simulink model "trabajo"  (R2021b)
settings: Solver=VariableStepAuto  StartTime=0.0  StopTime=1000  RelTol=1e-3
settings Model: Creator=david  LastModifiedBy=david

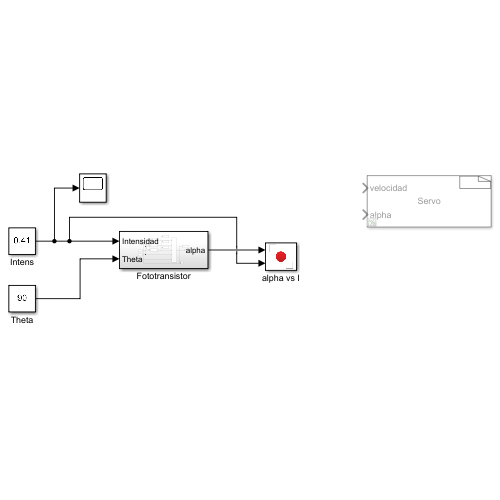
[thumbnail: Simulink's stored preview of the top-level diagram]
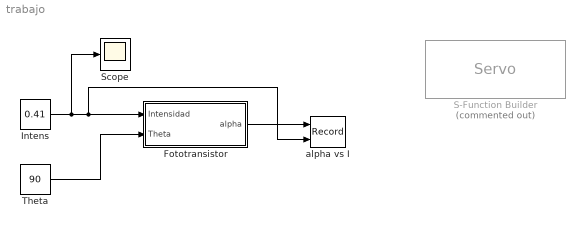
== system trabajo ==
  Fototransistor : Subsystem
  Intens : Constant  Value=0.41
  S-Function Builder : S-Function  Commented=on  FunctionName=Servo  SFunctionDeploymentMode=off  EnableBusSupport=off  mask(S-Function Builder){}
      mask help: Simulink:masks:SFunctionBuilder_MD
      mask init:
      | val = [[.9  0.75 0.75 1 1 .9 .9 1]',[1 1 0.75 0.75 .9 .9 1 .9]'];try , sys = get_param(gcb,'SfunBuilderFcnName');if isempty(sys), sys = get_param(gcb,'FunctionName'); end,catch, sys = get_param(gcb,'FunctionName'); end
      settings: CopyFcn=set_param(gcbh,'LinkStatus','none')  OpenFcn=sfunctionwizard(gcbh)
      mask Display: plot(val(:,1),val(:,2)),disp(sys),port_label('input',1,'velocidad'),port_label('input',2,'alpha')
  Scope : Scope
  Theta : Constant  Value=90
  alpha vs I : Record  FileSettingsInternal="{\"entries\":[{\"content\":{\"excelSettings\":{\"content\":{},\"type\":\"Streamout.ExcelSettings\"}},\"type\":\"Streamout.FileSettingStorage\",\"uuid\":\"fbcb0ebc-f8fb-453b-844a-01a15ffa13b0\"}],\"packageUris\":[\"http://schema.mathworks.com/mf0/streamout_blocks/R2020a\"],\"version\":\"1.0\"}"  Layout=[1 1]  SignalsInternal="{\"entries\":[{\"content\":{\"signals\":[{\"content\":{\"blockPath\":[\"trabajo/alpha vs I\"],\"channel\":[],\"dimensions\":[1],\"domain\":\"trabajo/alpha vs I\",\"lineColor\":\"#a2142f\",\"plots\":[1],\"port\":1,\"sid\":[\"\"],\"signalID\":274,\"signalName\":\"Fototransistor\"},\"type\":\"RecordBlkView.Signal\",\"uuid\":\"8a3e97ef-adf1-46c2-8f37-acfb5dae941a\"},{\"content\":{\"blockPath\":[\"trabajo/alpha vs I\"],\"channel\":[],\"dimensions\":[1],\"domain\":\"trabajo/alpha vs I\",\"lineColor\":\"#139fff\",\"plots\":[1],\"port\":2,\"sid\":[\"\"],\"signalID\":282,\"signalName\":\"Intens\"},\"type\":\"RecordBlkView.Signal\",\"uuid\":\"2784698f-795e-4f9a-a48f-a67caaf167da\"}]},\"type\":\"RecordBlkView.InputSignals\",\"uuid\":\"d232fc0d-a2d3-47a6-911d-820f8e91af49\"}],\"packageUris\":[\"http://schema.mathworks.com/mf0/streamout_blocks/R2020a\"],\"version\":\"1.0\"}"  VisualizationBindings="{\"xyplotplugin\":{\"info\":[{\"series\":[{\"bindingParametersList\":[{\"parameter\":\"X-Axis\",\"signalID\":274,\"signalName\":\"Fototransistor\"},{\"parameter\":\"Y-Axis\",\"signalID\":282,\"signalName\":\"Intens\"}],\"seriesID\":62877}],\"subplotID\":1}]}}"  CompatibilityTag=XY
  wires:
  Theta/1 -> Fototransistor/2(Theta)
  Fototransistor/1(alpha) -> alpha vs I/1
  Intens/1 -> Scope/1, alpha vs I/2, Fototransistor/1(Intensidad)

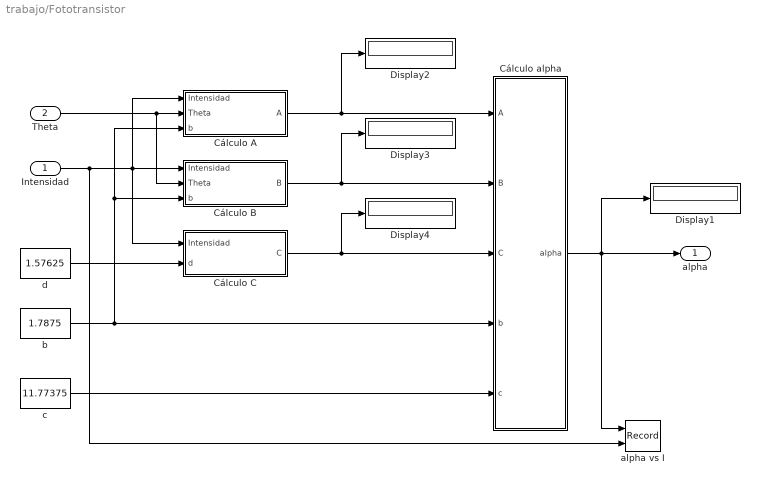
== system trabajo/Fototransistor ==
  Intensidad : Inport
  Theta : Inport  Port=2
  Cálculo A : Subsystem
  Cálculo B : Subsystem
  Cálculo C : Subsystem
  Cálculo alpha : MATLAB Function  TreatAsAtomicUnit=on
  Display{1..4} (4 alike) : Display
  alpha vs I : Record  FileSettingsInternal="{\"entries\":[{\"content\":{\"excelSettings\":{\"content\":{},\"type\":\"Streamout.ExcelSettings\"}},\"type\":\"Streamout.FileSettingStorage\",\"uuid\":\"38f66441-0a7a-4b0d-9ae6-422619585ecf\"}],\"packageUris\":[\"http://schema.mathworks.com/mf0/streamout_blocks/R2020a\"],\"version\":\"1.0\"}"  Layout=[1 1]  SignalsInternal="{\"entries\":[{\"content\":{\"signals\":[{\"content\":{\"blockPath\":[\"trabajo/Fototransistor/alpha vs I\"],\"channel\":[],\"dimensions\":[1],\"domain\":\"trabajo/Fototransistor/alpha vs I\",\"lineColor\":\"#a2142f\",\"plots\":[1],\"port\":1,\"sid\":[\"\"],\"signalID\":278,\"signalName\":\"Cálculo alpha\"},\"type\":\"RecordBlkView.Signal\",\"uuid\":\"1ab597ee-08d6-410f-8960-5a2a34f2bd90\"},{\"content\":{\"blockPath\":[\"trabajo/Fototransistor/alpha vs I\"],\"channel\":[],\"dimensions\":[1],\"domain\":\"trabajo/Fototransistor/alpha vs I\",\"lineColor\":\"#139fff\",\"plots\":[1],\"port\":2,\"sid\":[\"\"],\"signalID\":286,\"signalName\":\"Intensidad\"},\"type\":\"RecordBlkView.Signal\",\"uuid\":\"886f58e7-63e7-44eb-90ed-22280a59bf2c\"}]},\"type\":\"RecordBlkView.InputSignals\",\"uuid\":\"d4679059-a868-458c-b4b8-0854d651fb2d\"}],\"packageUris\":[\"http://schema.mathworks.com/mf0/streamout_blocks/R2020a\"],\"version\":\"1.0\"}"  VisualizationBindings="{\"xyplotplugin\":{\"info\":[{\"series\":[{\"bindingParametersList\":[{\"parameter\":\"X-Axis\",\"signalID\":278,\"signalName\":\"CÃ¡lculo alpha\"},{\"parameter\":\"Y-Axis\",\"signalID\":286,\"signalName\":\"Intensidad\"}],\"seriesID\":16912}],\"subplotID\":1}]}}"  CompatibilityTag=XY
  b : Constant  Value=1.7875
  c : Constant  Value=11.77375
  d : Constant  Value=1.57625
  alpha : Outport
  wires:
  Cálculo C/1(C) -> Display4/1, Cálculo alpha/3(C)
  Cálculo alpha/1(alpha) -> Display1/1, alpha/1, alpha vs I/1
  Intensidad/1 -> Cálculo B/1(Intensidad), Cálculo A/1(Intensidad), Cálculo C/1(Intensidad), alpha vs I/2
  Theta/1 -> Cálculo B/2(Theta), Cálculo A/2(Theta)
  Cálculo B/1(B) -> Display3/1, Cálculo alpha/2(B)
  Cálculo A/1(A) -> Display2/1, Cálculo alpha/1(A)
  b/1 -> Cálculo alpha/4(b), Cálculo B/3(b), Cálculo A/3(b)
  c/1 -> Cálculo alpha/5(c)
  d/1 -> Cálculo C/2(d)

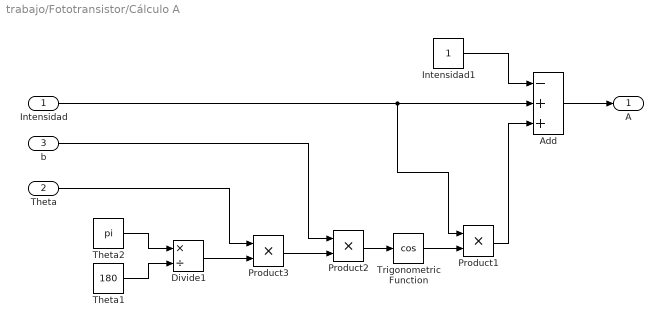
== system trabajo/Fototransistor/Cálculo A ==
  Intensidad : Inport
  Theta : Inport  Port=2
  b : Inport  Port=3
  Add : Sum  Inputs=-++
  Divide1 : Product  Inputs=*/
  Intensidad1 : Constant
  Product1 : Product
  Product2 : Product
  Product3 : Product
  Theta1 : Constant  Value=180
  Theta2 : Constant  Value=pi
  Trigonometric Function : Trigonometry  Operator=cos
  A : Outport
  wires:
  Divide1/1 -> Product3/2
  Product3/1 -> Product2/2
  Theta2/1 -> Divide1/1
  Intensidad1/1 -> Add/1
  Product1/1 -> Add/3
  Theta1/1 -> Divide1/2
  Trigonometric Function/1 -> Product1/2
  Product2/1 -> Trigonometric Function/1
  Intensidad/1 -> Product1/1, Add/2
  Theta/1 -> Product3/1
  Add/1 -> A/1
  b/1 -> Product2/1

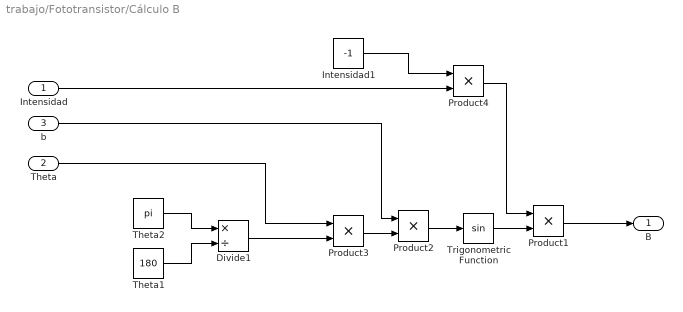
== system trabajo/Fototransistor/Cálculo B ==
  Intensidad : Inport
  Theta : Inport  Port=2
  b : Inport  Port=3
  Divide1 : Product  Inputs=*/
  Intensidad1 : Constant  Value=-1
  Product{1..4} (4 alike) : Product
  Theta1 : Constant  Value=180
  Theta2 : Constant  Value=pi
  Trigonometric Function : Trigonometry
  B : Outport
  wires:
  Divide1/1 -> Product3/2
  Product3/1 -> Product2/2
  Theta2/1 -> Divide1/1
  Product1/1 -> B/1
  Theta1/1 -> Divide1/2
  Trigonometric Function/1 -> Product1/2
  Product2/1 -> Trigonometric Function/1
  Intensidad/1 -> Product4/2
  Theta/1 -> Product3/1
  Intensidad1/1 -> Product4/1
  Product4/1 -> Product1/1
  b/1 -> Product2/1

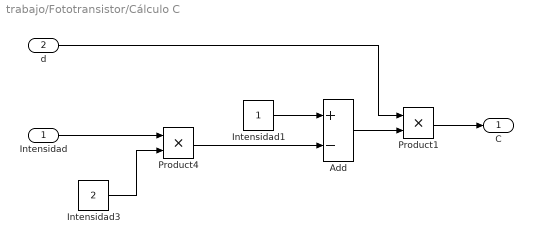
== system trabajo/Fototransistor/Cálculo C ==
  Intensidad : Inport
  d : Inport  Port=2
  Add : Sum  Inputs=+-
  Intensidad1 : Constant
  Intensidad3 : Constant  Value=2
  Product1 : Product
  Product4 : Product
  C : Outport
  wires:
  Intensidad1/1 -> Add/1
  Intensidad/1 -> Product4/1
  Intensidad3/1 -> Product4/2
  Product4/1 -> Add/2
  Add/1 -> Product1/2
  Product1/1 -> C/1
  d/1 -> Product1/1

== matlab function trabajo/Fototransistor/Cálculo alpha ==
  data: A input; alpha output; B input; C input; b input; c input
function alpha = fcn(A, B, C, b, c)

    if ((A+C ~= 0) && (-B*sqrt(A^2+B^2-C^2)+A^2+A*C+B^2 ~= 0))
        
        alpha = 2*atan((B-sqrt(A^2+B^2-C^2))/(A+C));

    elseif ((A+C ~= 0) && (B*sqrt(A^2+B^2-C^2)+A^2+A*C+B^2 ~= 0))

        alpha = 2*atan((B+sqrt(A^2+B^2-C^2))/(A+C));

    elseif ((B ~= 0) && (A^2+B^2~=0) && (C == -A))

        alpha = -2*atan(A/B);

    elseif (A == -C)

        alpha = pi;

    else

        alpha = 1000;

    end

    alpha = (alpha -c*pi/180)/b;

    alpha = alpha*180/pi;

end
